simulink model "takeoff"  (R2025b)
settings: Solver=ode4  StartTime=0.0  StopTime=150  FixedStep=0.001  RelTol=1e-3
values from neighbouring files (symbols this model uses):
  a0 = 340.294    [basedata.m]    (also in basedata.mat; control_design.mat; landing_init.m; landing_plan.mat)
  b_ref = 2.0    (= 2)    [basedata.m]    (also in basedata.mat; control_design.mat; landing_init.m; landing_plan.mat)
  c_gear = [0.8e4, 1.4e4, 1.4e4]    [basedata.m]    (also in basedata.mat = [8000 14000 14000]; control_design.mat = [8000 14000 14000]; landing_init.m; landing_plan.mat = [8000 14000 14000])
  c_lat = [1.4e4, 2.2e4, 2.2e4]    [basedata.m]    (also in basedata.mat = [14000 22000 22000]; control_design.mat = [14000 22000 22000]; landing_init.m; landing_plan.mat = [14000 22000 22000])
  c_ref = 0.9    [basedata.m]    (also in basedata.mat; control_design.mat; landing_init.m; landing_plan.mat)
  c_roll = [0.020, 0.018, 0.018]    [basedata.m]    (also in basedata.mat = [0.02 0.018 0.018]; control_design.mat = [0.02 0.018 0.018]; landing_init.m; landing_plan.mat = [0.02 0.018 0.018])
  CD0 = 0.045    [basedata.m]    (also in basedata.mat; canshujisuan.m; control_design.mat; landing_init.m)
  CL0 = 0.083    [basedata.m]    (also in basedata.mat; control_design.mat; landing_init.m; landing_plan.mat)
  CLa = 3.80    (= 3.8)    [basedata.m]    (also in basedata.mat; canshujisuan.m = 2.5; control_design.mat; landing_init.m)
  Clb = -0.08    [basedata.m]    (also in basedata.mat; control_design.mat; landing_init.m; landing_plan.mat)
  Clda = -0.20    (= -0.2)    [basedata.m]    (also in basedata.mat; control_design.mat; landing_init.m; landing_plan.mat)
  CLde = 0.28    [basedata.m]    (also in basedata.mat; control_design.mat; landing_init.m; landing_plan.mat)
  Clp = -0.70    (= -0.7)    [basedata.m]    (also in basedata.mat; control_design.mat; landing_init.m; landing_plan.mat)
  CLq = 4.50    (= 4.5)    [basedata.m]    (also in basedata.mat; canshujisuan.m = 3; control_design.mat; landing_init.m)
  Clr = 0.08    [basedata.m]    (also in basedata.mat; control_design.mat; landing_init.m; landing_plan.mat)
  Cm0 = 0.060    (= 0.06)    [basedata.m]    (also in basedata.mat; control_design.mat; landing_init.m; landing_plan.mat)
  Cma = -0.80    (= -0.8)    [basedata.m]    (also in basedata.mat; control_design.mat; landing_init.m; landing_plan.mat)
  Cmde = -0.90    (= -0.9)    [basedata.m]    (also in basedata.mat; control_design.mat; landing_init.m; landing_plan.mat)
  Cmq = -18.0    (= -18)    [basedata.m]    (also in basedata.mat; control_design.mat; landing_init.m; landing_plan.mat)
  Cnb = 0.25    [basedata.m]    (also in basedata.mat; control_design.mat; landing_init.m; landing_plan.mat)
  Cndr = -0.15    [basedata.m]    (also in basedata.mat; control_design.mat; landing_init.m; landing_plan.mat)
  Cnp = -0.04    [basedata.m]    (also in basedata.mat; control_design.mat; landing_init.m; landing_plan.mat)
  Cnr = -0.45    [basedata.m]    (also in basedata.mat; control_design.mat; landing_init.m; landing_plan.mat)
  CSb = -0.70    (= -0.7)    [basedata.m]    (also in basedata.mat; control_design.mat; landing_init.m; landing_plan.mat)
  CSdr = 0.18    [basedata.m]    (also in basedata.mat; control_design.mat; landing_init.m; landing_plan.mat)
  CSr = 0.12    [basedata.m]    (also in basedata.mat; control_design.mat; landing_init.m; landing_plan.mat)
  D = 0.5 * rho0 * V^2 * S_ref * CD_current    [canshujisuan.m]
  D0 = 1400    [basedata.m]    (also in basedata.mat; control_design.mat; landing.m; landing_init.m)
  da_max = 25    [basedata.m]    (also in basedata.mat; control_design.mat; landing_init.m; landing_plan.mat)
  da_min = -da_max    (= -25)    [basedata.m]    (also in basedata.mat; control_design.mat; landing_init.m; landing_plan.mat)
  de_max = 25    [basedata.m]    (also in basedata.mat; control_design.mat; landing_init.m; landing_plan.mat)
  de_min = -de_max    (= -25)    [basedata.m]    (also in basedata.mat; control_design.mat; landing_init.m; landing_plan.mat)
  DH = pi / 180    (= 0.0174532925199)    [basedata.m]    (also in basedata.mat; control_design.mat; landing_init.m; landing_plan.mat)
  dr_max = 25    [basedata.m]    (also in basedata.mat; control_design.mat; landing_init.m; landing_plan.mat)
  dr_min = -dr_max    (= -25)    [basedata.m]    (also in basedata.mat; control_design.mat; landing_init.m; landing_plan.mat)
  g = 9.80665    [basedata.m]    (also in basedata.mat; canshujisuan.m; control_design.mat; landing_init.m)
  gamma1 = -0.125844364415    [basedata.mat]    (also in landing_trajectory.m = asin(max(min(gamma1_arg, 1), -1)); landingplan.mat)
  gamma2 = -0.0261780104712    [basedata.mat]    (also in landing_trajectory.m = -0.0261799387799; landingplan.mat = 0.0261780104712)
  ground_z = 0.0    (= 0)    [basedata.m]    (also in basedata.mat; control_design.mat; landing_init.m; landing_plan.mat)
  HD = 180 / pi    (= 57.2957795131)    [basedata.m]    (also in basedata.mat; control_design.mat; landing_init.m; landing_plan.mat)
  I = [ Ixx, -Ixy, -Ixz ... (first row only)    [basedata.m]    (also in basedata.mat = [120  0  0; 0  480  0; 0  0  520]; control_design.mat = [120  0  0; 0  480  0; 0  0  520]; landing_init.m; landing_plan.mat = [120  0  0; 0  480  0; 0  0  520])
  K = 0.12    [basedata.m]    (also in basedata.mat; canshujisuan.m = 0.08; control_design.mat; landing_init.m)
  K_alpha = 7.5375    [basedata.mat]    (also in control_design.m = (((wd_pitch^2)-a24))/(2*kesi_pitch*wd_pitch); control_design.mat; controller.m = 5; landingplan.mat)
  k_gear = [1.0e5, 3.0e5, 3.0e5]    [basedata.m]    (also in basedata.mat = [100000 300000 300000]; control_design.mat = [100000 300000 300000]; landing_init.m; landing_plan.mat = [100000 300000 300000])
  Kn_pitch = -0.120095403309    [basedata.mat]    (also in control_design.m = -(2.2*g*(wd_pitch)^2)/(Tr*(((wd_pitch)^2)-a24)*V_control*a34; control_design.mat; controller.m = (2.2*wd^2*g)/(Tr*(wd^2-a24)*V_test*a34); landingplan.mat)
  Kw_pitch = -0.483749055178    [basedata.mat]    (also in control_design.m = -2*kesi_pitch*wd_pitch/a25; control_design.mat; controller.m = -(2*zeta*wd) / a25; landingplan.mat)
  m = 600.0    (= 600)    [basedata.m]    (also in basedata.mat; canshujisuan.m; control_design.mat; landing_init.m)
  mu_brake = [0.0, 0.55, 0.55]    [basedata.m]    (also in basedata.mat = [0 0.55 0.55]; control_design.mat = [0 0.55 0.55]; landing_init.m; landing_plan.mat = [0 0.55 0.55])
  phi0 = 0    [control_design.mat]    (also in landing.m; landing_init.m; landing_init.mat; landing_plan.mat)
  psi0 = 0    [control_design.mat]    (also in landing.m; landing_init.m; landing_init.mat; landing_plan.mat)
  r_left_b = r_gear_b(:,2)    [basedata.m]    (also in basedata.mat = [-0.333333333333 -0.8 0.65]; control_design.mat = [-0.333333333333 -0.8 0.65]; landing_init.m; landing_plan.mat = [-0.333333333333 -0.8 0.65])
  r_nose_b = r_gear_b(:,1)    [basedata.m]    (also in basedata.mat = [2 0 0.65]; control_design.mat = [2 0 0.65]; landing_init.m; landing_plan.mat = [2 0 0.65])
  r_right_b = r_gear_b(:,3)    [basedata.m]    (also in basedata.mat = [-0.333333333333 0.8 0.65]; control_design.mat = [-0.333333333333 0.8 0.65]; landing_init.m; landing_plan.mat = [-0.333333333333 0.8 0.65])
  rho0 = 1.225    [basedata.m]    (also in basedata.mat; canshujisuan.m; control_design.mat; landing_init.m)
  S_ref = 1.2    [basedata.m]    (also in basedata.mat; canshujisuan.m; control_design.mat; landing_init.m)
  theta0 = 0.0523560209424    [control_design.mat]    (also in landing.m = 0; landing_init.m; landing_init.mat = 0.0523598775598; landing_plan.mat)
  u0_b = 128    [control_design.mat]    (also in landing.m; landing_init.m; landing_init.mat = 100; landing_plan.mat)
  v0_b = 0    [control_design.mat]    (also in landing.m; landing_init.m; landing_init.mat; landing_plan.mat)
  v_eps = 0.20    (= 0.2)    [basedata.m]    (also in basedata.mat; control_design.mat; landing_init.m; landing_plan.mat)
  V_min = 3    [control_design.mat]    (also in landing.m; landing_init.m; landing_plan.mat; landingplan.mat)
  w0_b = 0    [control_design.mat]    (also in landing.m; landing_init.m; landing_init.mat; landing_plan.mat)
  wheel_radius = 0.18    [basedata.m]    (also in basedata.mat; control_design.mat; landing_init.m; landing_plan.mat)
  WOW_on = 0.000    (= 0)    [basedata.m]    (also in basedata.mat; control_design.mat; landing_init.m; landing_plan.mat)
  Xg0 = -12000    [control_design.mat]    (also in landing.m; landing_init.m; landing_init.mat = -8000; landing_plan.mat)
  Yg0 = 0    [control_design.mat]    (also in landing.m; landing_init.m; landing_init.mat; landing_plan.mat)
  Zg0 = ground_z - wheel_radius - r_gear_b(3,1) + static_deflection    [basedata.m]    (also in basedata.mat = -0.8215943; control_design.mat = -1000; landing.m = -1000; landing_init.m = -1000)
undefined symbols (not defined in the file or in its folder): I_xz, I_yz, Ix_Iy, Iy_Iz, Iz_Ix
libraries: simulink x52, matrix_library x19
(part 1 of 4)
settings Model: SimulationMode=accelerator  Creator=34355  LastModifiedBy=fjy

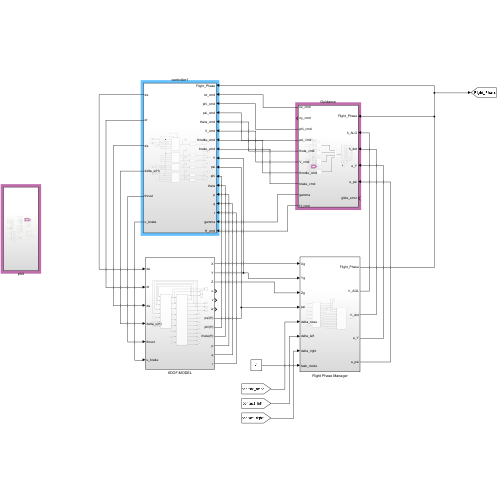
[thumbnail: Simulink's stored preview of the top-level diagram]
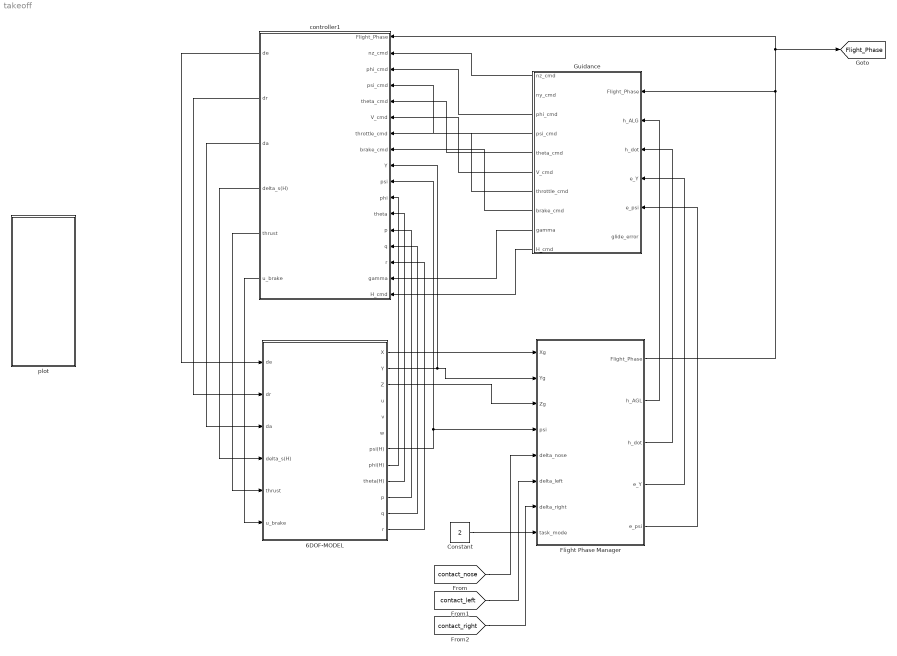
== system takeoff ==
  6DOF-MODEL : Subsystem
  Constant : Constant  Value=2
  Flight Phase Manager : Subsystem
  Guidance : Subsystem
  controller1 : Subsystem
  plot : Subsystem
  tag scope: Flight_Phase=global
  wires:
  Constant/1 -> Flight Phase Manager/8(task_mode)
  6DOF-MODEL/1(X) -> Flight Phase Manager/1(Xg)
  6DOF-MODEL/2(Y) -> Flight Phase Manager/2(Yg), controller1/9(Y)
  6DOF-MODEL/3(Z) -> Flight Phase Manager/3(Zg)
  6DOF-MODEL/7(psi(H)) -> controller1/10(psi), Flight Phase Manager/4(psi)
  [contact_nose] -> Flight Phase Manager/5(delta_nose)
  [contact_left] -> Flight Phase Manager/6(delta_left)
  [contact_right] -> Flight Phase Manager/7(delta_right)
  Flight Phase Manager/1(Flight_Phase) -> controller1/1(Flight_Phase), [Flight_Phase], Guidance/1(Flight_Phase)
  Flight Phase Manager/2(h_AGL) -> Guidance/2(h_ALG)
  Flight Phase Manager/3(h_dot) -> Guidance/3(h_dot)
  Flight Phase Manager/4(e_Y) -> Guidance/4(e_Y)
  Flight Phase Manager/5(e_psi) -> Guidance/5(e_psi)
  Guidance/1(nz_cmd) -> controller1/2(nz_cmd)
  Guidance/3(phi_cmd) -> controller1/3(phi_cmd)
  Guidance/4(psi_cmd) -> controller1/4(psi_cmd)
  Guidance/5(theta_cmd) -> controller1/5(theta_cmd)
  Guidance/6(V_cmd) -> controller1/6(V_cmd)
  Guidance/7(throttle_cmd) -> controller1/7(throttle_cmd)
  Guidance/8(brake_cmd) -> controller1/8(brake_cmd)
  6DOF-MODEL/8(phi(H)) -> controller1/11(phi)
  6DOF-MODEL/9(theta(H)) -> controller1/12(theta)
  6DOF-MODEL/10(p) -> controller1/13(p)
  6DOF-MODEL/11(q) -> controller1/14(q)
  6DOF-MODEL/12(r) -> controller1/15(r)
  controller1/1(de) -> 6DOF-MODEL/1(de)
  controller1/2(dr) -> 6DOF-MODEL/2(dr)
  controller1/3(da) -> 6DOF-MODEL/3(da)
  controller1/4(delta_s(H)) -> 6DOF-MODEL/4(delta_s(H))
  controller1/5(thrust) -> 6DOF-MODEL/5(thrust)
  controller1/6(u_brake) -> 6DOF-MODEL/6(u_brake)
  Guidance/9(gamma) -> controller1/16(gamma)
  Guidance/10(H_cmd) -> controller1/17(H_cmd)

== system takeoff/6DOF-MODEL ==
  de : Inport
  dr : Inport  Port=2
  da : Inport  Port=3
  delta_s(H) : Inport  Port=4
  thrust : Inport  Port=5
  u_brake : Inport  Port=6
  AERO-PARAMETER : Subsystem
  Scope : Scope
      settings: ActiveDisplayYMinimum=1.1177  ActiveDisplayYMaximum=6.98546
  Scope5 : Scope
      settings: ActiveDisplayYMinimum=-8256.02255  ActiveDisplayYMaximum=5856.30436
  Scope6 : Scope
      settings: ActiveDisplayYMinimum=-1607.05651  ActiveDisplayYMaximum=178.56183  DataLoggingVariableName=ScopeData4
  动力学 : Subsystem
  X : Outport
  Y : Outport  Port=2
  Z : Outport  Port=3
  u : Outport  Port=4
  v : Outport  Port=5
  w : Outport  Port=6
  psi(H) : Outport  Port=7
  phi(H) : Outport  Port=8
  theta(H) : Outport  Port=9
  p : Outport  Port=10
  q : Outport  Port=11
  r : Outport  Port=12
  wires:
  动力学/1(alpha(D)) -> Scope/1, AERO-PARAMETER/1(alpha(D))
  thrust/1 -> 动力学/7(thrust)
  u_brake/1 -> 动力学/9(u_brake)
  AERO-PARAMETER/1(D) -> Scope6/1, 动力学/1(D)
  AERO-PARAMETER/2(L) -> Scope5/1, 动力学/2(L)
  AERO-PARAMETER/3(S) -> 动力学/3(S)
  AERO-PARAMETER/4(MX) -> 动力学/4(MX)
  AERO-PARAMETER/5(MY) -> 动力学/5(MY)
  AERO-PARAMETER/6(MZ) -> 动力学/6(MZ)
  delta_s(H)/1 -> 动力学/8(delta_s(H))
  动力学/2(beta(D)) -> AERO-PARAMETER/2(beta(D))
  动力学/3(p) -> p/1, AERO-PARAMETER/3(p(H))
  动力学/4(q) -> q/1, AERO-PARAMETER/4(q(H))
  动力学/5(r) -> r/1, AERO-PARAMETER/5(r(H))
  de/1 -> AERO-PARAMETER/6(de(D))
  dr/1 -> AERO-PARAMETER/7(dr(D))
  da/1 -> AERO-PARAMETER/8(da)
  动力学/14(w) -> w/1
  动力学/7(Y) -> Y/1
  动力学/8(Z) -> Z/1
  动力学/13(v) -> v/1
  动力学/11(psi(H)) -> psi(H)/1
  动力学/12(u) -> u/1
  动力学/10(theta(H)) -> theta(H)/1
  动力学/6(X) -> X/1
  动力学/9(phi(H)) -> phi(H)/1

== system takeoff/Flight Phase Manager ==
  Xg : Inport
  Yg : Inport  Port=2
  Zg : Inport  Port=3
  psi : Inport  Port=4
  delta_nose : Inport  Port=5
  delta_left : Inport  Port=6
  delta_right : Inport  Port=7
  task_mode : Inport  Port=8
  Data Pre-processing : Subsystem
  Phase Logic : Stateflow chart  TreatAsAtomicUnit=on
  Flight_Phase : Outport
  h_AGL : Outport  Port=2
  h_dot : Outport  Port=3
  e_Y : Outport  Port=4
  e_psi : Outport  Port=5
  wires:
  Xg/1 -> Data Pre-processing/1(Xg)
  Yg/1 -> Data Pre-processing/2(Yg)
  Zg/1 -> Data Pre-processing/3(Zg)
  psi/1 -> Data Pre-processing/4(psi)
  delta_nose/1 -> Data Pre-processing/5(delta_nose)
  delta_left/1 -> Data Pre-processing/6(delta_left)
  delta_right/1 -> Data Pre-processing/7(delta_right)
  Phase Logic/1(Flight_Phase) -> Flight_Phase/1
  task_mode/1 -> Phase Logic/13(Task_Mode)
  Data Pre-processing/1(h_AGL) -> h_AGL/1, Phase Logic/1(h_AGL)
  Data Pre-processing/2(V_runway) -> Phase Logic/2(V_runway)
  Data Pre-processing/3(h_dot) -> h_dot/1, Phase Logic/3(h_dot)
  Data Pre-processing/6(nose_on_ground) -> Phase Logic/4(nose_on_ground)
  Data Pre-processing/7(main_on_ground) -> Phase Logic/5(main_on_ground)
  Data Pre-processing/8(airborne) -> Phase Logic/6(airborne)
  Data Pre-processing/9(reach_VR) -> Phase Logic/7(reach_VR)
  Data Pre-processing/10(safe_climb) -> Phase Logic/8(safe_climb)
  Data Pre-processing/11(localizer_captured) -> Phase Logic/9(localizer_captured)
  Data Pre-processing/12(glideslope_captured) -> Phase Logic/10(glideslope_captured)
  Data Pre-processing/13(flare_entry) -> Phase Logic/11(flare_entry)
  Data Pre-processing/14(stop_condition) -> Phase Logic/12(stop_condition)
  Data Pre-processing/4(e_Y) -> e_Y/1
  Data Pre-processing/5(e_psi) -> e_psi/1

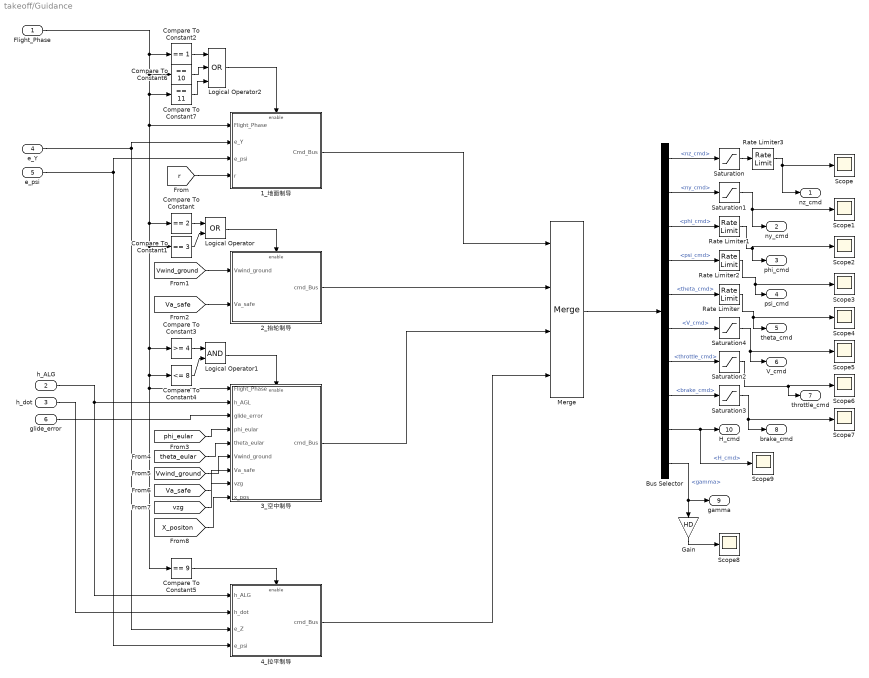
== system takeoff/Guidance ==
  Flight_Phase : Inport
  h_ALG : Inport  Port=2
  h_dot : Inport  Port=3
  e_Y : Inport  Port=4
  e_psi : Inport  Port=5
  glide_error : Inport  Port=6
  1_地面制导 : Subsystem
  "2_抬轮制导 " : Subsystem
  3_空中制导 : Subsystem
  4_拉平制导 : Subsystem
  Bus Selector : BusSelector  OutputSignals=nz_cmd,ny_cmd,phi_cmd,psi_cmd,theta_cmd,V_cmd,throttle_cmd,brake_cmd,H_cmd,gamma
  Compare To Constant : simulink/Logic and Bit Operations/Compare To Constant  relop===  const=2  OutDataTypeStr=boolean
  Compare To Constant1 : simulink/Logic and Bit Operations/Compare To Constant  relop===  const=3  OutDataTypeStr=boolean
  Compare To Constant2 : simulink/Logic and Bit Operations/Compare To Constant  relop===  const=1  OutDataTypeStr=boolean
  Compare To Constant3 : simulink/Logic and Bit Operations/Compare To Constant  relop=>=  const=4  OutDataTypeStr=boolean
  Compare To Constant4 : simulink/Logic and Bit Operations/Compare To Constant  relop=<=  const=8  OutDataTypeStr=boolean
  Compare To Constant5 : simulink/Logic and Bit Operations/Compare To Constant  relop===  const=9  OutDataTypeStr=boolean
  Compare To Constant6 : simulink/Logic and Bit Operations/Compare To Constant  relop===  const=10  OutDataTypeStr=boolean
  Compare To Constant7 : simulink/Logic and Bit Operations/Compare To Constant  relop===  const=11  OutDataTypeStr=boolean
  Gain : Gain  Gain=HD
  Logical Operator : Logic  Operator=OR  AllPortsSameDT=off  OutDataTypeStr=boolean
  Logical Operator1 : Logic  AllPortsSameDT=off  OutDataTypeStr=boolean
  Logical Operator2 : Logic  Operator=OR  Inputs=3  AllPortsSameDT=off  OutDataTypeStr=boolean
  Merge : Merge  Inputs=4
  Rate Limiter : RateLimiter  RisingSlewLimit=1*DH  FallingSlewLimit=-1*DH  SampleTimeMode=inherited
  Rate Limiter1 : RateLimiter  RisingSlewLimit=10*DH  FallingSlewLimit=-10*DH  SampleTimeMode=inherited
  Rate Limiter2 : RateLimiter  RisingSlewLimit=10*DH  FallingSlewLimit=-10*DH  SampleTimeMode=inherited
  Rate Limiter3 : RateLimiter  RisingSlewLimit=0.8  FallingSlewLimit=-0.8  SampleTimeMode=inherited
  Saturation : Saturate  UpperLimit=2  LowerLimit=-2
  Saturation1 : Saturate  UpperLimit=2  LowerLimit=-2
  Saturation2 : Saturate  UpperLimit=1  LowerLimit=0
  Saturation3 : Saturate  UpperLimit=1  LowerLimit=0
  Saturation4 : Saturate  UpperLimit=250  LowerLimit=0
  Scope{,1..9} (10 alike) : Scope
      Scope settings: ActiveDisplayYMinimum=-0.19965  ActiveDisplayYMaximum=1.13329  DataLoggingVariableName=ScopeData2
      Scope1 settings: ActiveDisplayYMinimum=-0.00301  ActiveDisplayYMaximum=0.00493  DataLoggingVariableName=ScopeData3
      Scope2 settings: ActiveDisplayYMinimum=-1  ActiveDisplayYMaximum=1  DataLoggingVariableName=ScopeData4
      Scope3 settings: ActiveDisplayYMinimum=-0.0909  ActiveDisplayYMaximum=0.01814  DataLoggingVariableName=ScopeData5
      Scope4 settings: ActiveDisplayYMinimum=-0.02618  ActiveDisplayYMaximum=0.23562  DataLoggingVariableName=ScopeData6
      Scope5 settings: DataLoggingVariableName=ScopeData7
      Scope6 settings: DataLoggingVariableName=ScopeData8
      Scope7 settings: DataLoggingVariableName=ScopeData9
      Scope8 settings: ActiveDisplayYMinimum=-8.111644826033606  ActiveDisplayYMaximum=0.90129386955928936
      Scope9 settings: ActiveDisplayYMinimum=-113.79263048910924  ActiveDisplayYMaximum=1137.202950532841  DataLoggingVariableName=ScopeData25
  nz_cmd : Outport
  ny_cmd : Outport  Port=2
  phi_cmd : Outport  Port=3
  psi_cmd : Outport  Port=4
  theta_cmd : Outport  Port=5
  V_cmd : Outport  Port=6
  throttle_cmd : Outport  Port=7
  brake_cmd : Outport  Port=8
  gamma : Outport  Port=9
  H_cmd : Outport  Port=10
  wires:
  Flight_Phase/1 -> Compare To Constant6/1, Compare To Constant7/1, 1_地面制导/1(Flight_Phase), Compare To Constant3/1, Compare To Constant4/1, Compare To Constant5/1, 3_空中制导/1(Flight_Phase), Compare To Constant1/1, Compare To Constant/1, Compare To Constant2/1
  e_Y/1 -> 1_地面制导/2(e_Y), 4_拉平制导/3(e_Z)
  Merge/1 -> Bus Selector/1
  e_psi/1 -> 1_地面制导/3(e_psi), 4_拉平制导/4(e_psi)
  h_ALG/1 -> 4_拉平制导/1(h_ALG), 3_空中制导/2(h_AGL)
  h_dot/1 -> 4_拉平制导/2(h_dot)
  glide_error/1 -> 3_空中制导/3(glide_error)
  Saturation1/1 -> ny_cmd/1, Scope1/1
  Compare To Constant/1 -> Logical Operator/1
  Compare To Constant1/1 -> Logical Operator/2
  Logical Operator/1 -> "2_抬轮制导 "/Enable
  Compare To Constant3/1 -> Logical Operator1/1
  Compare To Constant4/1 -> Logical Operator1/2
  Logical Operator1/1 -> 3_空中制导/Enable
  Compare To Constant5/1 -> 4_拉平制导/Enable
  Compare To Constant2/1 -> Logical Operator2/1
  Compare To Constant6/1 -> Logical Operator2/2
  Compare To Constant7/1 -> Logical Operator2/3
  Logical Operator2/1 -> 1_地面制导/Enable
  Rate Limiter/1 -> theta_cmd/1, Scope4/1
  Rate Limiter1/1 -> phi_cmd/1, Scope2/1
  1_地面制导/1(Cmd_Bus) -> Merge/1
  "2_抬轮制导 "/1(cmd_Bus) -> Merge/2
  3_空中制导/1(cmd_Bus) -> Merge/3
  4_拉平制导/1(cmd_Bus) -> Merge/4
  Rate Limiter2/1 -> psi_cmd/1, Scope3/1
  Saturation3/1 -> brake_cmd/1, Scope7/1
  Saturation4/1 -> V_cmd/1, Scope5/1
  Saturation/1 -> Rate Limiter3/1
  Rate Limiter3/1 -> nz_cmd/1, Scope/1
  Saturation2/1 -> throttle_cmd/1, Scope6/1
  [r] -> 1_地面制导/4(r)
  [Vwind_ground] -> "2_抬轮制导 "/1(Vwind_ground)
  [Va_safe] -> "2_抬轮制导 "/2(Va_safe)
  [phi_eular] -> 3_空中制导/4(phi_eular)
  [theta_eular] -> 3_空中制导/5(theta_eular)
  [Vwind_ground] -> 3_空中制导/6(Vwind_ground)
  [Va_safe] -> 3_空中制导/7(Va_safe)
  Bus Selector/1 -> Saturation/1  "<nz_cmd>"
  Bus Selector/2 -> Saturation1/1  "<ny_cmd>"
  Bus Selector/3 -> Rate Limiter1/1  "<phi_cmd>"
  Bus Selector/4 -> Rate Limiter2/1  "<psi_cmd>"
  Bus Selector/5 -> Rate Limiter/1  "<theta_cmd>"
  Bus Selector/6 -> Saturation4/1  "<V_cmd>"
  Bus Selector/7 -> Saturation2/1  "<throttle_cmd>"
  Bus Selector/8 -> Saturation3/1  "<brake_cmd>"
  [vzg] -> 3_空中制导/8(vzg)
  [X_positon] -> 3_空中制导/9(x_pos)
  Bus Selector/10 -> Gain/1, gamma/1  "<gamma>"
  Bus Selector/9 -> Scope9/1, H_cmd/1  "<H_cmd>"
  Gain/1 -> Scope8/1

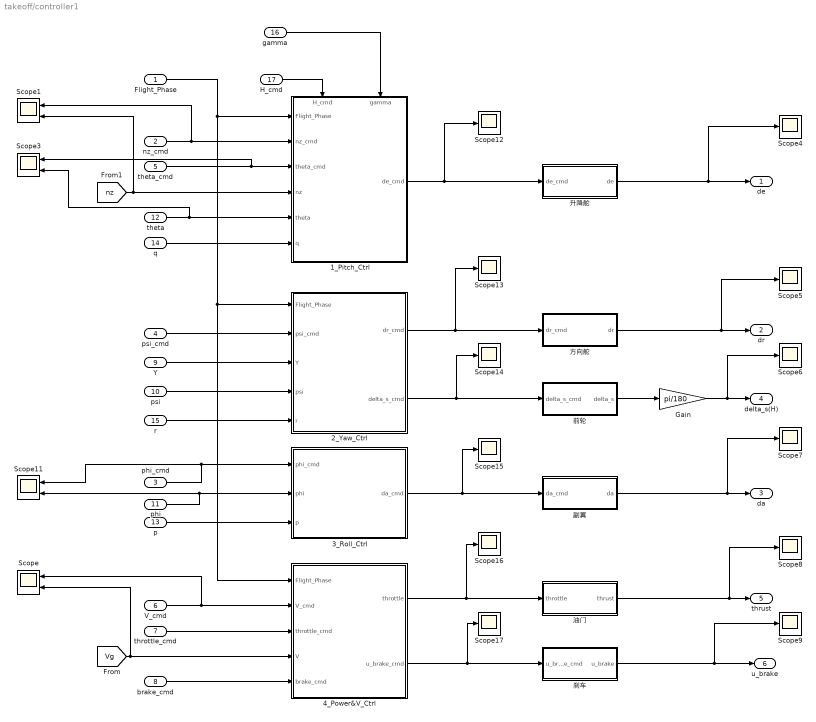
== system takeoff/controller1 ==
  Flight_Phase : Inport
  nz_cmd : Inport  Port=2
  phi_cmd : Inport  Port=3
  psi_cmd : Inport  Port=4
  theta_cmd : Inport  Port=5
  V_cmd : Inport  Port=6
  throttle_cmd : Inport  Port=7
  brake_cmd : Inport  Port=8
  Y : Inport  Port=9
  psi : Inport  Port=10
  phi : Inport  Port=11
  theta : Inport  Port=12
  p : Inport  Port=13
  q : Inport  Port=14
  r : Inport  Port=15
  gamma : Inport  Port=16
  H_cmd : Inport  Port=17
  1_Pitch_Ctrl : Subsystem
      settings: PortSchema="{\"entries\":[{\"content\":{\"sides\":[{\"content\":{\"connectorIds\":[\"In1\",\"In2\",\"In3\",\"In4\",\"In5\",\"In6\"]},\"type\":\"ConnectorPlacement.EquallySpacedRectSide\",\"uuid\":\"27d13232-9f89-4ac1-9c77-5758657de7c7\"},{\"content\":{\"connectorIds\":[\"Out1\"],\"side\":\"RIGHT\"},\"type\":\"ConnectorPlacement.EquallySpacedRectSide\",\"uuid\":\"ae62ad8c-a405-4422-b5ec-9ac723f70591\"},{\"content\":{\"connectorIds\":[\"In7\",\"In8\"],\"side\":\"TOP\"},\"type\":\"ConnectorPlacement.EquallySpacedRectSide\",\"uuid\":\"4cebe0f4-d768-4fb6-931c-2fd4183255b7\"}]},\"type\":\"ConnectorPlacement.EquallySpacedConnector\",\"uuid\":\"2c44e0df-7f94-4dab-9232-216c905b911f\"}],\"packageUris\":[\"http://schema.mathworks.com/mf0/Connector/R2020b\"],\"version\":\"1.0\"}"
  2_Yaw_Ctrl : Subsystem
  3_Roll_Ctrl : Subsystem
  4_Power&V_Ctrl : Subsystem
  Gain : Gain  Gain=pi/180
  Scope{,1,3,11} (4 alike) : Scope  NumInputPorts=2
      Scope settings: ActiveDisplayYMinimum=-25.14963  ActiveDisplayYMaximum=226.34663  DataLoggingVariableName=ScopeData3
      Scope1 settings: ActiveDisplayYMinimum=-0.22546  ActiveDisplayYMaximum=1.36559  DataLoggingVariableName=ScopeData7
      Scope11 settings: ActiveDisplayYMinimum=-0.00059  ActiveDisplayYMaximum=0.00038  DataLoggingVariableName=ScopeData2
      Scope3 settings: ActiveDisplayYMinimum=-0.02682  ActiveDisplayYMaximum=0.23988  DataLoggingVariableName=ScopeData10
  Scope{4..9,12..17} (12 alike) : Scope
      Scope12 settings: ActiveDisplayYMinimum=-14.28559  ActiveDisplayYMaximum=7.54847
      Scope13 settings: ActiveDisplayYMinimum=-7.28617  ActiveDisplayYMaximum=15.25402  DataLoggingVariableName=ScopeData2
      Scope14 settings: ActiveDisplayYMinimum=-0.00117  ActiveDisplayYMaximum=0.0105  DataLoggingVariableName=ScopeData3
      Scope15 settings: ActiveDisplayYMinimum=-0.22974  ActiveDisplayYMaximum=1.237  DataLoggingVariableName=ScopeData4
      Scope16 settings: ActiveDisplayYMinimum=0.24658  ActiveDisplayYMaximum=1.08371  DataLoggingVariableName=ScopeData5
      Scope17 settings: ActiveDisplayYMinimum=-1  ActiveDisplayYMaximum=1  DataLoggingVariableName=ScopeData6
      Scope4 settings: ActiveDisplayYMinimum=-13.80049  ActiveDisplayYMaximum=6.51267  DataLoggingVariableName=ScopeData11
      Scope5 settings: ActiveDisplayYMinimum=-7.23665  ActiveDisplayYMaximum=15.24812
      Scope6 settings: ActiveDisplayYMinimum=-2E-5  ActiveDisplayYMaximum=0.00018  DataLoggingVariableName=ScopeData2
      Scope7 settings: ActiveDisplayYMinimum=-0.15917  ActiveDisplayYMaximum=1.07702  DataLoggingVariableName=ScopeData3
      Scope8 settings: ActiveDisplayYMinimum=-375  ActiveDisplayYMaximum=3375  DataLoggingVariableName=ScopeData4
      Scope9 settings: ActiveDisplayYMinimum=-1  ActiveDisplayYMaximum=1  DataLoggingVariableName=ScopeData5
  刹车 : Subsystem
  前轮 : Subsystem
  副翼 : Subsystem
  升降舵 : Subsystem
  方向舵 : Subsystem
  油门 : Subsystem
  de : Outport
  dr : Outport  Port=2
  da : Outport  Port=3
  delta_s(H) : Outport  Port=4
  thrust : Outport  Port=5
  u_brake : Outport  Port=6
  wires:
  phi_cmd/1 -> Scope11/1, 3_Roll_Ctrl/1(phi_cmd)
  phi/1 -> Scope11/2, 3_Roll_Ctrl/2(phi)
  p/1 -> 3_Roll_Ctrl/3(p)
  brake_cmd/1 -> 4_Power&V_Ctrl/5(brake_cmd)
  4_Power&V_Ctrl/1(throttle) -> 油门/1(throttle), Scope16/1
  Flight_Phase/1 -> 1_Pitch_Ctrl/1(Flight_Phase), 2_Yaw_Ctrl/1(Flight_Phase), 4_Power&V_Ctrl/1(Flight_Phase)
  nz_cmd/1 -> Scope1/1, 1_Pitch_Ctrl/2(nz_cmd)
  psi_cmd/1 -> 2_Yaw_Ctrl/2(psi_cmd)
  [nz] -> Scope1/2, 1_Pitch_Ctrl/4(nz)
  q/1 -> 1_Pitch_Ctrl/6(q)
  V_cmd/1 -> Scope/1, 4_Power&V_Ctrl/2(V_cmd)
  [Vg] -> Scope/2, 4_Power&V_Ctrl/4(V)
  Gain/1 -> Scope6/1, delta_s(H)/1
  theta_cmd/1 -> Scope3/1, 1_Pitch_Ctrl/3(theta_cmd)
  1_Pitch_Ctrl/1(de_cmd) -> 升降舵/1(de_cmd), Scope12/1
  2_Yaw_Ctrl/1(dr_cmd) -> Scope13/1, 方向舵/1(dr_cmd)
  2_Yaw_Ctrl/2(delta_s_cmd) -> Scope14/1, 前轮/1(delta_s_cmd)
  3_Roll_Ctrl/1(da_cmd) -> Scope15/1, 副翼/1(da_cmd)
  4_Power&V_Ctrl/2(u_brake_cmd) -> 刹车/1(u_brake_cmd), Scope17/1
  theta/1 -> Scope3/2, 1_Pitch_Ctrl/5(theta)
  throttle_cmd/1 -> 4_Power&V_Ctrl/3(throttle_cmd)
  Y/1 -> 2_Yaw_Ctrl/3(Y)
  psi/1 -> 2_Yaw_Ctrl/4(psi)
  r/1 -> 2_Yaw_Ctrl/5(r)
  升降舵/1(de) -> Scope4/1, de/1
  方向舵/1(dr) -> Scope5/1, dr/1
  前轮/1(delta_s) -> Gain/1
  副翼/1(da) -> Scope7/1, da/1
  油门/1(thrust) -> Scope8/1, thrust/1
  刹车/1(u_brake) -> Scope9/1, u_brake/1
  H_cmd/1 -> 1_Pitch_Ctrl/7(H_cmd)
  gamma/1 -> 1_Pitch_Ctrl/8(gamma)

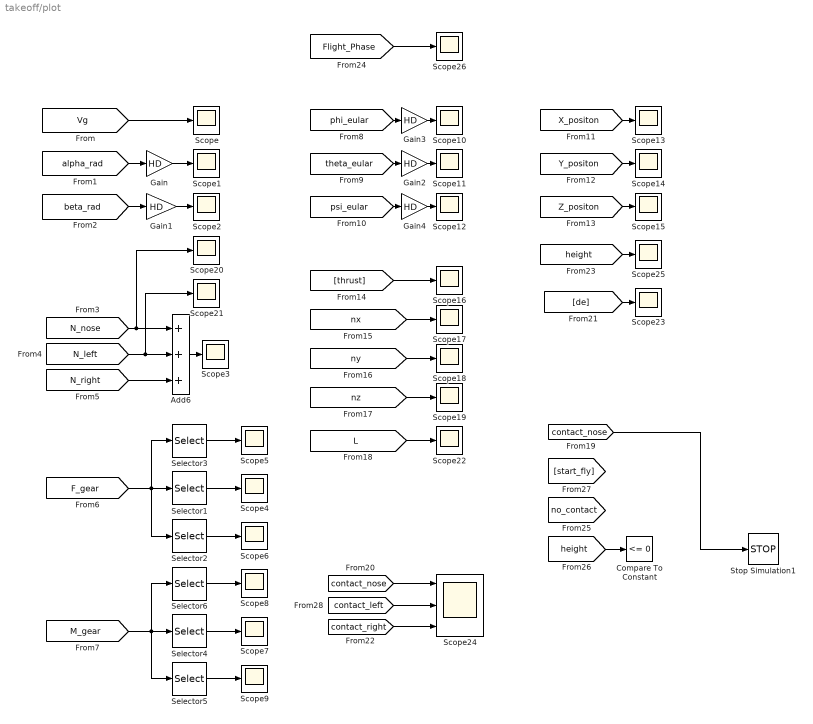
== system takeoff/plot ==
  Add6 : Sum  Inputs=+++
  Compare To Constant : simulink/Logic and Bit Operations/Compare To Constant  relop=<=  const=0  OutDataTypeStr=boolean
  Gain{,1..4} (5 alike) : Gain  Gain=HD
  Scope{,1..23,25..26} (26 alike) : Scope
      Scope settings: ActiveDisplayYMinimum=118.60732407894886  ActiveDisplayYMaximum=211.43694512925961
      Scope1 settings: ActiveDisplayYMinimum=-66.97288  ActiveDisplayYMaximum=12.39263  DataLoggingVariableName=ScopeData2
      Scope10 settings: ActiveDisplayYMinimum=-0.02449  ActiveDisplayYMaximum=0.1104  DataLoggingVariableName=ScopeData12
      Scope11 settings: ActiveDisplayYMinimum=-8.03156734153454  ActiveDisplayYMaximum=9.991113407153664  DataLoggingVariableName=ScopeData13
      Scope12 settings: ActiveDisplayYMinimum=-2.0624  ActiveDisplayYMaximum=0.22916  DataLoggingVariableName=ScopeData14
      Scope13 settings: ActiveDisplayYMinimum=-457.52925  ActiveDisplayYMaximum=4117.76325  DataLoggingVariableName=ScopeData15
      Scope14 settings: ActiveDisplayYMinimum=-1.79752  ActiveDisplayYMaximum=0.19975  DataLoggingVariableName=ScopeData16
      Scope15 settings: ActiveDisplayYMinimum=-1124.98258  ActiveDisplayYMaximum=124.08518  DataLoggingVariableName=ScopeData17
      Scope16 settings: ActiveDisplayYMinimum=1428.28526  ActiveDisplayYMaximum=3174.63497  DataLoggingVariableName=ScopeData18
      Scope17 settings: ActiveDisplayYMinimum=-0.69402  ActiveDisplayYMaximum=5.48306  DataLoggingVariableName=ScopeData19
      Scope18 settings: ActiveDisplayYMinimum=-1  ActiveDisplayYMaximum=1  DataLoggingVariableName=ScopeData20
      Scope19 settings: ActiveDisplayYMinimum=-1.39533  ActiveDisplayYMaximum=-0.75578  DataLoggingVariableName=ScopeData21
      Scope2 settings: ActiveDisplayYMinimum=-0.24043  ActiveDisplayYMaximum=0.0115  DataLoggingVariableName=ScopeData3
      Scope20 settings: ActiveDisplayYMinimum=-109.07344  ActiveDisplayYMaximum=981.66096  DataLoggingVariableName=ScopeData2
      Scope21 settings: ActiveDisplayYMinimum=-315.21375  ActiveDisplayYMaximum=2836.92375  DataLoggingVariableName=ScopeData5
      Scope22 settings: ActiveDisplayYMinimum=-1.39533  ActiveDisplayYMaximum=-0.75578  DataLoggingVariableName=ScopeData5
      Scope23 settings: ActiveDisplayYMinimum=-4.93736  ActiveDisplayYMaximum=28.32637
      Scope25 settings: ActiveDisplayYMinimum=-125.13549679187696  ActiveDisplayYMaximum=1136.7614641690736
      Scope26 settings: ActiveDisplayYMinimum=5.75  ActiveDisplayYMaximum=8.25  DataLoggingVariableName=ScopeData4
      Scope3 settings: ActiveDisplayYMinimum=-6.8710410861604161E+86  ActiveDisplayYMaximum=6.1839369775443757E+87  DataLoggingVariableName=ScopeData4
      Scope4 settings: ActiveDisplayYMinimum=-1  ActiveDisplayYMaximum=1  DataLoggingVariableName=ScopeData6
      Scope5 settings: ActiveDisplayYMinimum=-126.98754  ActiveDisplayYMaximum=57.45616  DataLoggingVariableName=ScopeData7
      Scope6 settings: ActiveDisplayYMinimum=-6622.10957  ActiveDisplayYMaximum=735.78995  DataLoggingVariableName=ScopeData8
      Scope7 settings: ActiveDisplayYMinimum=5883.9899999999234  ActiveDisplayYMaximum=5883.99000000002  DataLoggingVariableName=ScopeData9
      Scope8 settings: ActiveDisplayYMinimum=-1  ActiveDisplayYMaximum=1  DataLoggingVariableName=ScopeData10
      Scope9 settings: ActiveDisplayYMinimum=-1  ActiveDisplayYMaximum=1  DataLoggingVariableName=ScopeData11
  Scope24 : Scope  NumInputPorts=3
      settings: ActiveDisplayYMinimum=-0.125  ActiveDisplayYMaximum=1.125  DataLoggingVariableName=ScopeData6
  Selector1 : Selector  InputPortWidth=3  IndexOptions=Index vector (dialog)  Indices=2  OutputSizes=1
  Selector2 : Selector  InputPortWidth=3  IndexOptions=Index vector (dialog)  Indices=3  OutputSizes=1
  Selector3 : Selector  InputPortWidth=3  IndexOptions=Index vector (dialog)  Indices=1  OutputSizes=1
  Selector4 : Selector  InputPortWidth=3  IndexOptions=Index vector (dialog)  Indices=2  OutputSizes=1
  Selector5 : Selector  InputPortWidth=3  IndexOptions=Index vector (dialog)  Indices=3  OutputSizes=1
  Selector6 : Selector  InputPortWidth=3  IndexOptions=Index vector (dialog)  Indices=1  OutputSizes=1
  Stop Simulation1 : Stop
  wires:
  [N_nose] -> Add6/1, Scope20/1
  [N_left] -> Scope21/1, Add6/2
  [N_right] -> Add6/3
  [Vg] -> Scope/1
  [alpha_rad] -> Gain/1
  [beta_rad] -> Gain1/1
  Add6/1 -> Scope3/1
  Selector3/1 -> Scope5/1
  Selector2/1 -> Scope6/1
  Selector1/1 -> Scope4/1
  [F_gear] -> Selector2/1, Selector1/1, Selector3/1
  Selector6/1 -> Scope8/1
  Selector4/1 -> Scope7/1
  [M_gear] -> Selector6/1, Selector4/1, Selector5/1
  Selector5/1 -> Scope9/1
  [psi_eular] -> Gain4/1
  [theta_eular] -> Gain2/1
  [phi_eular] -> Gain3/1
  Gain1/1 -> Scope2/1
  Gain/1 -> Scope1/1
  Gain2/1 -> Scope11/1
  [Y_positon] -> Scope14/1
  [X_positon] -> Scope13/1
  [Z_positon] -> Scope15/1
  Gain3/1 -> Scope10/1
  Gain4/1 -> Scope12/1
  [thrust] -> Scope16/1
  [nx] -> Scope17/1
  [ny] -> Scope18/1
  [nz] -> Scope19/1
  [L] -> Scope22/1
  [de] -> Scope23/1
  [contact_nose] -> Stop Simulation1/1
  [height] -> Scope25/1
  [height] -> Compare To Constant/1
  [contact_nose] -> Scope24/1
  [contact_left] -> Scope24/2
  [contact_right] -> Scope24/3
  [Flight_Phase] -> Scope26/1

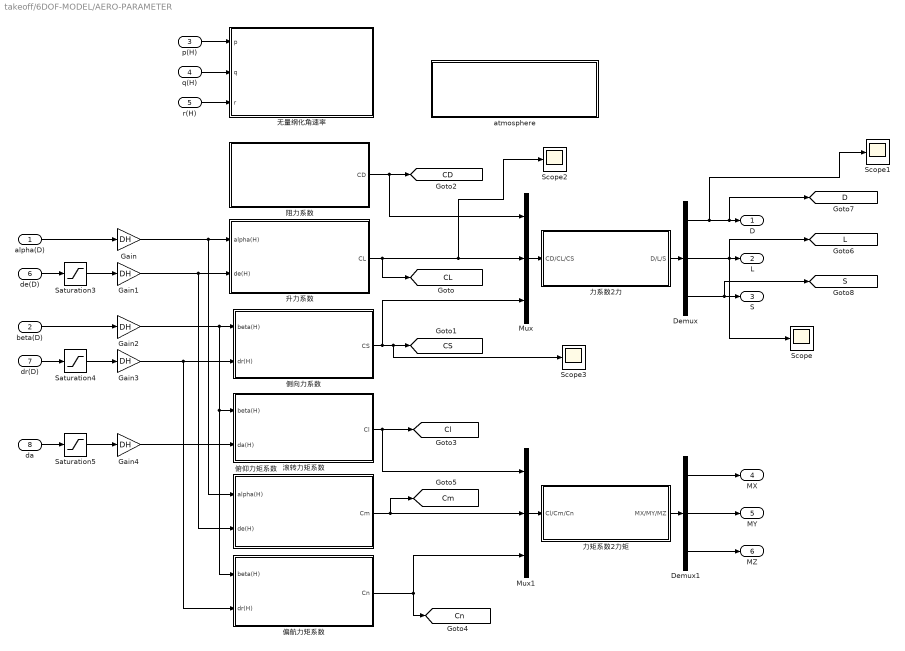
== system takeoff/6DOF-MODEL/AERO-PARAMETER ==
  alpha(D) : Inport
  beta(D) : Inport  Port=2
  p(H) : Inport  Port=3
  q(H) : Inport  Port=4
  r(H) : Inport  Port=5
  de(D) : Inport  Port=6
  dr(D) : Inport  Port=7
  da : Inport  Port=8
  Demux : Demux  Outputs=3
  Demux1 : Demux  Outputs=3
  Gain{,1..4} (5 alike) : Gain  Gain=DH
  Mux : Mux  Inputs=3
  Mux1 : Mux  Inputs=3
  Saturation3 : Saturate  UpperLimit=de_max  LowerLimit=de_min
  Saturation4 : Saturate  UpperLimit=dr_max  LowerLimit=dr_min
  Saturation5 : Saturate  UpperLimit=da_max  LowerLimit=da_min
  Scope{,1..3} (4 alike) : Scope
      Scope settings: ActiveDisplayYMinimum=-8344.45381  ActiveDisplayYMaximum=927.16153  DataLoggingVariableName=ScopeData20
      Scope1 settings: ActiveDisplayYMinimum=568.90057  ActiveDisplayYMaximum=1072.36921  DataLoggingVariableName=ScopeData24
      Scope2 settings: ActiveDisplayYMinimum=-7.3517  ActiveDisplayYMaximum=7.03431  DataLoggingVariableName=ScopeData2
      Scope3 settings: ActiveDisplayYMinimum=-0.27324  ActiveDisplayYMaximum=0.20902  DataLoggingVariableName=ScopeData2
  atmosphere : Subsystem
  侧向力系数 : Subsystem
  俯仰力矩系数 : Subsystem
  偏航力矩系数 : Subsystem
  力矩系数2力矩 : Subsystem
  力系数2力 : Subsystem
  升力系数 : Subsystem
  无量纲化角速率 : Subsystem
  滚转力矩系数 : Subsystem
  阻力系数 : Subsystem
  D : Outport
  L : Outport  Port=2
  S : Outport  Port=3
  MX : Outport  Port=4
  MY : Outport  Port=5
  MZ : Outport  Port=6
  tag scope: CD=global, CL=global, CS=global, Cl=global, Cm=global, Cn=global, D=global, L=global, S=global
  wires:
  升力系数/1(CL) -> [CL], Scope2/1, Mux/2
  侧向力系数/1(CS) -> Mux/3, Scope3/1, [CS]
  da/1 -> Saturation5/1
  Saturation5/1 -> Gain4/1
  Saturation4/1 -> Gain3/1
  dr(D)/1 -> Saturation4/1
  de(D)/1 -> Saturation3/1
  Saturation3/1 -> Gain1/1
  beta(D)/1 -> Gain2/1
  alpha(D)/1 -> Gain/1
  Gain/1 -> 升力系数/1(alpha(H)), 俯仰力矩系数/1(alpha(H))
  Gain1/1 -> 升力系数/2(de(H)), 俯仰力矩系数/2(de(H))
  Gain2/1 -> 侧向力系数/1(beta(H)), 偏航力矩系数/1(beta(H)), 滚转力矩系数/1(beta(H))
  Gain3/1 -> 侧向力系数/2(dr(H)), 偏航力矩系数/2(dr(H))
  Gain4/1 -> 滚转力矩系数/2(da(H))
  p(H)/1 -> 无量纲化角速率/1(p)
  q(H)/1 -> 无量纲化角速率/2(q)
  r(H)/1 -> 无量纲化角速率/3(r)
  阻力系数/1(CD) -> Mux/1, [CD]
  滚转力矩系数/1(Cl) -> [Cl], Mux1/1
  俯仰力矩系数/1(Cm) -> Mux1/2, [Cm]
  偏航力矩系数/1(Cn) -> [Cn], Mux1/3
  Mux/1 -> 力系数2力/1(CD/CL/CS)
  Mux1/1 -> 力矩系数2力矩/1(Cl/Cm/Cn)
  Demux/2 -> Scope/1, [L], L/1
  力系数2力/1(D/L/S) -> Demux/1
  Demux/1 -> Scope1/1, [D], D/1
  Demux/3 -> [S], S/1
  力矩系数2力矩/1(MX/MY/MZ) -> Demux1/1
  Demux1/1 -> MX/1
  Demux1/2 -> MY/1
  Demux1/3 -> MZ/1

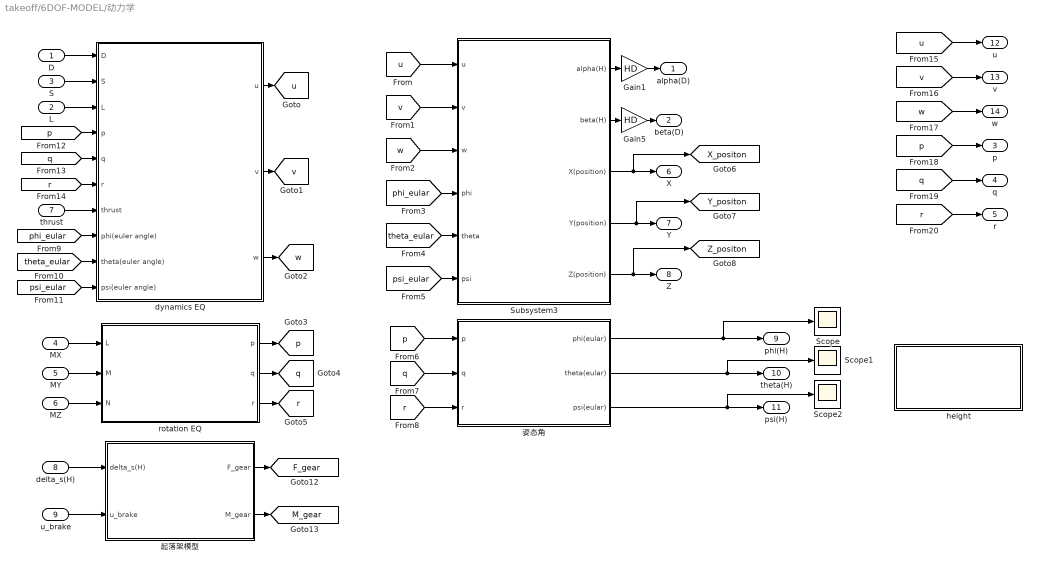
== system takeoff/6DOF-MODEL/动力学 ==
  D : Inport
  L : Inport  Port=2
  S : Inport  Port=3
  MX : Inport  Port=4
  MY : Inport  Port=5
  MZ : Inport  Port=6
  thrust : Inport  Port=7
  delta_s(H) : Inport  Port=8
  u_brake : Inport  Port=9
  Gain1 : Gain  Gain=HD
  Gain5 : Gain  Gain=HD
  Scope : Scope
      settings: ActiveDisplayYMinimum=-1  ActiveDisplayYMaximum=1  DataLoggingVariableName=ScopeData4
  Scope1 : Scope
      settings: ActiveDisplayYMinimum=-57.279  ActiveDisplayYMaximum=136.57236  DataLoggingVariableName=ScopeData5
  Scope2 : Scope
      settings: ActiveDisplayYMinimum=-12.64721  ActiveDisplayYMaximum=113.82488  DataLoggingVariableName=ScopeData6
  Subsystem3 : Subsystem
  dynamics EQ : Subsystem
  height : Subsystem
  rotation EQ : Subsystem
  姿态角 : Subsystem
  起落架模型 : Subsystem
  alpha(D) : Outport
  beta(D) : Outport  Port=2
  p : Outport  Port=3
  q : Outport  Port=4
  r : Outport  Port=5
  X : Outport  Port=6
  Y : Outport  Port=7
  Z : Outport  Port=8
  phi(H) : Outport  Port=9
  theta(H) : Outport  Port=10
  psi(H) : Outport  Port=11
  u : Outport  Port=12
  v : Outport  Port=13
  w : Outport  Port=14
  tag scope: F_gear=global, M_gear=global, X_positon=global, Y_positon=global, Z_positon=global, p=global, q=global, r=global, u=global, v=global, w=global
  wires:
  姿态角/1(phi(eular)) -> Scope/1, phi(H)/1
  姿态角/2(theta(eular)) -> theta(H)/1, Scope1/1
  姿态角/3(psi(eular)) -> psi(H)/1, Scope2/1
  Gain5/1 -> beta(D)/1
  Gain1/1 -> alpha(D)/1
  [u] -> u/1
  [v] -> v/1
  [w] -> w/1
  [p] -> p/1
  [q] -> q/1
  [r] -> r/1
  起落架模型/1(F_gear) -> [F_gear]
  起落架模型/2(M_gear) -> [M_gear]
  MX/1 -> rotation EQ/1(L)
  MY/1 -> rotation EQ/2(M)
  MZ/1 -> rotation EQ/3(N)
  D/1 -> dynamics EQ/1(D)
  S/1 -> dynamics EQ/2(S)
  L/1 -> dynamics EQ/3(L)
  [p] -> dynamics EQ/4(p)
  [q] -> dynamics EQ/5(q)
  [r] -> dynamics EQ/6(r)
  thrust/1 -> dynamics EQ/7(thrust)
  [phi_eular] -> dynamics EQ/8(phi(euler angle))
  [theta_eular] -> dynamics EQ/9(theta(euler angle))
  [psi_eular] -> dynamics EQ/10(psi(euler angle))
  dynamics EQ/1(u) -> [u]
  dynamics EQ/2(v) -> [v]
  dynamics EQ/3(w) -> [w]
  [u] -> Subsystem3/1(u)
  [v] -> Subsystem3/2(v)
  [w] -> Subsystem3/3(w)
  [phi_eular] -> Subsystem3/4(phi)
  [theta_eular] -> Subsystem3/5(theta)
  [psi_eular] -> Subsystem3/6(psi)
  Subsystem3/1(alpha(H)) -> Gain1/1
  Subsystem3/2(beta(H)) -> Gain5/1
  Subsystem3/3(X(position)) -> [X_positon], X/1
  Subsystem3/4(Y(position)) -> [Y_positon], Y/1
  Subsystem3/5(Z(position)) -> [Z_positon], Z/1
  delta_s(H)/1 -> 起落架模型/1(delta_s(H))
  u_brake/1 -> 起落架模型/2(u_brake)
  rotation EQ/1(p) -> [p]
  rotation EQ/2(q) -> [q]
  rotation EQ/3(r) -> [r]
  [p] -> 姿态角/1(p)
  [q] -> 姿态角/2(q)
  [r] -> 姿态角/3(r)

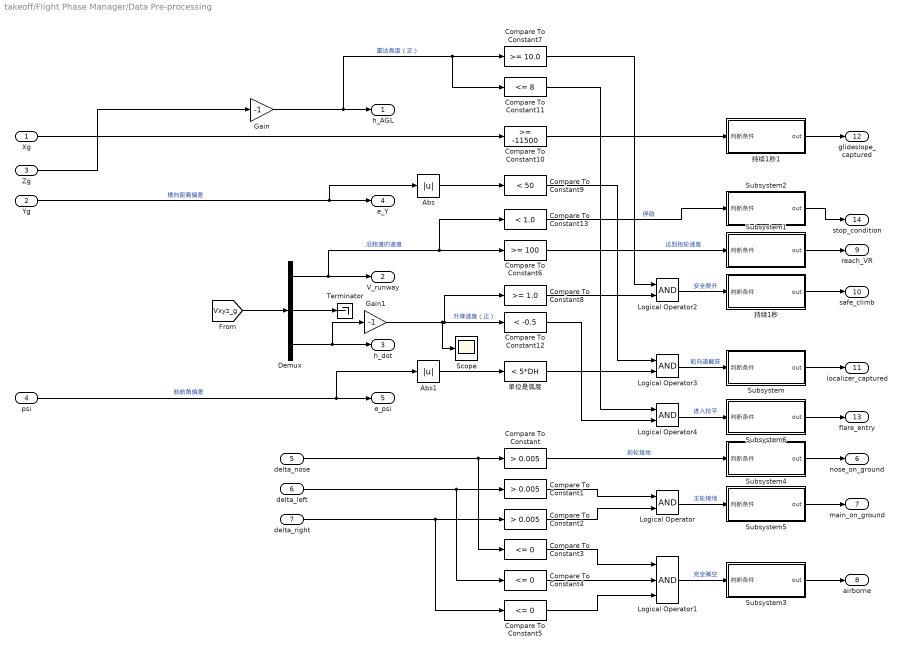
== system takeoff/Flight Phase Manager/Data Pre-processing ==
  Xg : Inport
  Yg : Inport  Port=2
  Zg : Inport  Port=3
  psi : Inport  Port=4
  delta_nose : Inport  Port=5
  delta_left : Inport  Port=6
  delta_right : Inport  Port=7
  Abs : Abs  SaturateOnIntegerOverflow=off
  Abs1 : Abs  SaturateOnIntegerOverflow=off
  Compare To Constant : simulink/Logic and Bit Operations/Compare To Constant  relop=>  const=0.005  OutDataTypeStr=boolean
  Compare To Constant1 : simulink/Logic and Bit Operations/Compare To Constant  relop=>  const=0.005  OutDataTypeStr=boolean
  Compare To Constant10 : simulink/Logic and Bit Operations/Compare To Constant  relop=>=  const=-11500  OutDataTypeStr=boolean
  Compare To Constant11 : simulink/Logic and Bit Operations/Compare To Constant  relop=<=  const=8  OutDataTypeStr=boolean
  Compare To Constant12 : simulink/Logic and Bit Operations/Compare To Constant  relop=<  const=-0.5  OutDataTypeStr=boolean
  Compare To Constant13 : simulink/Logic and Bit Operations/Compare To Constant  relop=<  const=1.0  OutDataTypeStr=boolean
  Compare To Constant2 : simulink/Logic and Bit Operations/Compare To Constant  relop=>  const=0.005  OutDataTypeStr=boolean
  Compare To Constant3 : simulink/Logic and Bit Operations/Compare To Constant  relop=<=  const=0  OutDataTypeStr=boolean
  Compare To Constant4 : simulink/Logic and Bit Operations/Compare To Constant  relop=<=  const=0  OutDataTypeStr=boolean
  Compare To Constant5 : simulink/Logic and Bit Operations/Compare To Constant  relop=<=  const=0  OutDataTypeStr=boolean
  Compare To Constant6 : simulink/Logic and Bit Operations/Compare To Constant  relop=>=  const=100  OutDataTypeStr=boolean
  Compare To Constant7 : simulink/Logic and Bit Operations/Compare To Constant  relop=>=  const=10.0  OutDataTypeStr=boolean
  Compare To Constant8 : simulink/Logic and Bit Operations/Compare To Constant  relop=>=  const=1.0  OutDataTypeStr=boolean
  Compare To Constant9 : simulink/Logic and Bit Operations/Compare To Constant  relop=<  const=50  OutDataTypeStr=boolean
  Demux : Demux  Outputs=3
  Gain : Gain  Gain=-1
  Gain1 : Gain  Gain=-1
  Logical Operator{,2..4} (4 alike) : Logic  AllPortsSameDT=off  OutDataTypeStr=boolean
  Logical Operator1 : Logic  Inputs=3  AllPortsSameDT=off  OutDataTypeStr=boolean
  Scope : Scope
      settings: ActiveDisplayYMinimum=-23.10985  ActiveDisplayYMaximum=40.49102  DataLoggingVariableName=ScopeData5
  Subsystem : Subsystem
  Subsystem1 : Subsystem
  Subsystem2 : Subsystem
  Subsystem3 : Subsystem
  Subsystem4 : Subsystem
  Subsystem5 : Subsystem
  Subsystem6 : Subsystem
  Terminator : Terminator
  单位是弧度 : simulink/Logic and Bit Operations/Compare To Constant  relop=<  const=5*DH  OutDataTypeStr=boolean
  持续1秒 : Subsystem
  持续1秒1 : Subsystem
  h_AGL : Outport
  V_runway : Outport  Port=2
  h_dot : Outport  Port=3
  e_Y : Outport  Port=4
  e_psi : Outport  Port=5
  nose_on_ground : Outport  Port=6
  main_on_ground : Outport  Port=7
  airborne : Outport  Port=8
  reach_VR : Outport  Port=9
  safe_climb : Outport  Port=10
  localizer_captured : Outport  Port=11
  glideslope_captured : Outport  Port=12
  flare_entry : Outport  Port=13
  stop_condition : Outport  Port=14
  wires:
  [Vxyz_g] -> Demux/1
  Demux/1 -> V_runway/1, Compare To Constant13/1, Compare To Constant6/1  "沿跑道的速度"
  psi/1 -> e_psi/1, Abs1/1  "航航角偏差"
  delta_nose/1 -> Compare To Constant3/1, Compare To Constant/1
  delta_left/1 -> Compare To Constant1/1, Compare To Constant4/1
  delta_right/1 -> Compare To Constant2/1, Compare To Constant5/1
  Compare To Constant1/1 -> Logical Operator/1
  Compare To Constant2/1 -> Logical Operator/2
  Compare To Constant4/1 -> Logical Operator1/2
  Compare To Constant3/1 -> Logical Operator1/1
  Compare To Constant5/1 -> Logical Operator1/3
  Compare To Constant8/1 -> Logical Operator2/2
  Compare To Constant7/1 -> Logical Operator2/1
  Abs/1 -> Compare To Constant9/1
  Abs1/1 -> 单位是弧度/1
  单位是弧度/1 -> Logical Operator3/2
  Compare To Constant9/1 -> Logical Operator3/1
  Compare To Constant11/1 -> Logical Operator4/1
  Compare To Constant12/1 -> Logical Operator4/2
  持续1秒/1(out) -> safe_climb/1
  Logical Operator3/1 -> Subsystem/1(判断条件)  "航向道截获"
  Subsystem/1(out) -> localizer_captured/1
  Logical Operator2/1 -> 持续1秒/1(判断条件)  "安全爬升"
  持续1秒1/1(out) -> glideslope_captured/1
  Subsystem1/1(out) -> reach_VR/1
  Compare To Constant6/1 -> Subsystem1/1(判断条件)  "达到抬轮速度"
  Subsystem2/1(out) -> stop_condition/1
  Compare To Constant13/1 -> Subsystem2/1(判断条件)  "停稳"
  Logical Operator1/1 -> Subsystem3/1(判断条件)  "完全腾空"
  Subsystem3/1(out) -> airborne/1
  Subsystem4/1(out) -> nose_on_ground/1
  Compare To Constant/1 -> Subsystem4/1(判断条件)  "前轮接地"
  Subsystem5/1(out) -> main_on_ground/1
  Logical Operator/1 -> Subsystem5/1(判断条件)  "主轮接地"
  Subsystem6/1(out) -> flare_entry/1
  Logical Operator4/1 -> Subsystem6/1(判断条件)  "进入拉平"
  Zg/1 -> Gain/1
  Yg/1 -> e_Y/1, Abs/1  "横向距离偏差"
  Gain/1 -> h_AGL/1, Compare To Constant7/1, Compare To Constant11/1  "雷达高度（正）"
  Gain1/1 -> Scope/1, Compare To Constant8/1, Compare To Constant12/1  "升降速度（正）"
  Demux/2 -> Terminator/1
  Demux/3 -> Gain1/1, h_dot/1
  Compare To Constant10/1 -> 持续1秒1/1(判断条件)
  Xg/1 -> Compare To Constant10/1

== system takeoff/Guidance/1_地面制导 ==
  Flight_Phase : Inport
  e_Y : Inport  Port=2
  e_psi : Inport  Port=3
  r : Inport  Port=4
  Enable : EnablePort
  Bus Creator : BusCreator  Inputs=10
  Compare To Constant1 : simulink/Logic and Bit Operations/Compare To Constant  relop===  const=11  OutDataTypeStr=boolean
  Constant : Constant  Value=0
  Constant3 : Constant
  Gain : Gain  Gain=-1
  Gain2 : Gain  Gain=0.08
  Gain3 : Gain  Gain=-0.85
  Gain4 : Gain  Gain=-0.2
  H_cmd : Constant  Value=0
  Sum : Sum  Inputs=|++
  Sum1 : Sum  Inputs=|++
  Switch1 : Switch  Criteria=u2 > Threshold  SaturateOnIntegerOverflow=off  InputSameDT=off
  V_cmd : Constant  Value=0
  gamma : Constant  Value=0
  ny_cmd : Constant  Value=0.0
  nz_cmd : Constant  Value=1.0
  phi_cmd : Constant  Value=0.0
  psi_cmd : Saturate  UpperLimit=25*pi/180  LowerLimit=-25*pi/180
  theta_cmd : Constant  Value=0.0
  throttle_cmd : Constant
  Cmd_Bus : Outport
  wires:
  Flight_Phase/1 -> Compare To Constant1/1
  Compare To Constant1/1 -> Switch1/2
  Constant3/1 -> Switch1/1
  Constant/1 -> Switch1/3
  nz_cmd/1 -> Bus Creator/1  "nz_cmd"
  ny_cmd/1 -> Bus Creator/2  "ny_cmd"
  phi_cmd/1 -> Bus Creator/3  "phi_cmd"
  psi_cmd/1 -> Bus Creator/4  "psi_cmd"
  theta_cmd/1 -> Bus Creator/5  "theta_cmd"
  Switch1/1 -> Bus Creator/8  "brake_cmd"
  Bus Creator/1 -> Cmd_Bus/1
  e_Y/1 -> Gain/1
  throttle_cmd/1 -> Bus Creator/7  "throttle_cmd"
  Gain/1 -> Gain2/1
  e_psi/1 -> Gain3/1
  Gain2/1 -> Sum/1
  Gain3/1 -> Sum/2
  Sum/1 -> Sum1/1
  Gain4/1 -> Sum1/2
  Sum1/1 -> psi_cmd/1
  V_cmd/1 -> Bus Creator/6  "V_cmd"
  r/1 -> Gain4/1
  gamma/1 -> Bus Creator/9  "gamma"
  H_cmd/1 -> Bus Creator/10  "H_cmd"

== system takeoff/Guidance/2_抬轮制导  ==
  Vwind_ground : Inport
  Va_safe : Inport  Port=2
  Enable : EnablePort  StatesWhenEnabling=reset
  Asin : Trigonometry  Operator=asin
  Bus Creator : BusCreator  Inputs=10
  Constant : Constant  Value=12
  Constant1 : Constant  Value=0
  Divide : Product  Inputs=*/
  Gain : Gain  Gain=DH
  Gain1 : Gain  Gain=-1
  H_cmd : Constant  Value=0
  Saturation2 : Saturate  UpperLimit=10*DH  LowerLimit=-10*DH
  Selector : Selector  InputPortWidth=3  IndexOptions=Index vector (dialog)  Indices=2  OutputSizes=1
  V_cmd : Constant  Value=200
  gamma : Constant  Value=0
  ny_cmd : Constant  Value=0
  nz_cmd : Constant
  phi_cmd : Constant  Value=0
  throttle_cmd : Constant
  cmd_Bus : Outport  InitialOutput=0
  wires:
  Constant1/1 -> Bus Creator/8  "brake_cmd"
  Saturation2/1 -> Bus Creator/4  "psi_cmd"
  V_cmd/1 -> Bus Creator/6  "V_cmd"
  throttle_cmd/1 -> Bus Creator/7  "throttle_cmd"
  nz_cmd/1 -> Bus Creator/1  "nz_cmd"
  Gain/1 -> Bus Creator/5  "theta_cmd"
  ny_cmd/1 -> Bus Creator/2  "ny_cmd"
  Bus Creator/1 -> cmd_Bus/1
  phi_cmd/1 -> Bus Creator/3  "phi_cmd"
  Constant/1 -> Gain/1
  Gain1/1 -> Saturation2/1
  Selector/1 -> Divide/1
  Divide/1 -> Asin/1
  Asin/1 -> Gain1/1
  Va_safe/1 -> Divide/2
  Vwind_ground/1 -> Selector/1
  H_cmd/1 -> Bus Creator/10  "H_cmd"
  gamma/1 -> Bus Creator/9  "gamma"

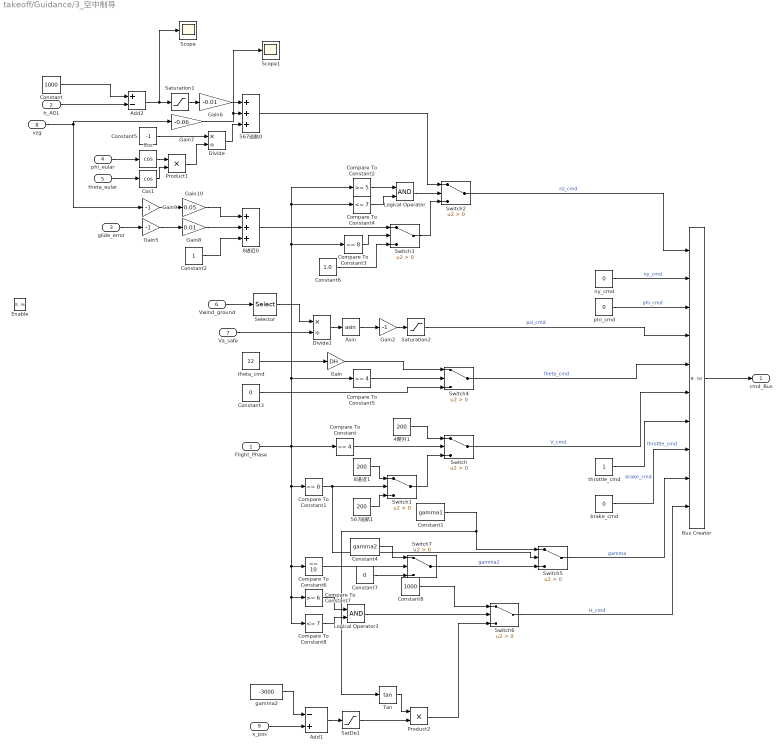
== system takeoff/Guidance/3_空中制导 ==
  Flight_Phase : Inport
  h_AGL : Inport  Port=2
  glide_error : Inport  Port=3
  phi_eular : Inport  Port=4
  theta_eular : Inport  Port=5
  Vwind_ground : Inport  Port=6
  Va_safe : Inport  Port=7
  vzg : Inport  Port=8
  x_pos : Inport  Port=9
  Enable : EnablePort
  4爬升1 : Constant  Value=200
  567巡航0 : Sum  Inputs=+++
  567巡航1 : Constant  Value=200
  8进近0 : Sum  Inputs=+++
  8进近1 : Constant  Value=200
  Add1 : Sum  Inputs=-+
  Add2 : Sum  Inputs=+-
  Asin : Trigonometry  Operator=asin
  Bus Creator : BusCreator  Inputs=10
  Compare To Constant : simulink/Logic and Bit Operations/Compare To Constant  relop===  const=4  OutDataTypeStr=boolean
  Compare To Constant1 : simulink/Logic and Bit Operations/Compare To Constant  relop===  const=8  OutDataTypeStr=boolean
  Compare To Constant2 : simulink/Logic and Bit Operations/Compare To Constant  relop=>=  const=5  OutDataTypeStr=boolean
  Compare To Constant3 : simulink/Logic and Bit Operations/Compare To Constant  relop===  const=8  OutDataTypeStr=boolean
  Compare To Constant4 : simulink/Logic and Bit Operations/Compare To Constant  relop=<=  const=7  OutDataTypeStr=boolean
  Compare To Constant5 : simulink/Logic and Bit Operations/Compare To Constant  relop===  const=4  OutDataTypeStr=boolean
  Compare To Constant6 : simulink/Logic and Bit Operations/Compare To Constant  relop===  const=10  OutDataTypeStr=boolean
  Compare To Constant7 : simulink/Logic and Bit Operations/Compare To Constant  relop=>=  const=6  OutDataTypeStr=boolean
  Compare To Constant8 : simulink/Logic and Bit Operations/Compare To Constant  relop=<=  const=7  OutDataTypeStr=boolean
  Constant : Constant  Value=1000
  Constant1 : Constant  Value=gamma1
  Constant2 : Constant
  Constant3 : Constant  Value=0
  Constant4 : Constant  Value=gamma2
  Constant5 : Constant  Value=-1
  Constant6 : Constant  Value=1.0
  Constant7 : Constant  Value=0
  Constant8 : Constant  Value=1000
  Cos : Trigonometry  Operator=cos
  Cos1 : Trigonometry  Operator=cos
  Divide : Product  Inputs=*/
  Divide1 : Product  Inputs=*/
  Gain : Gain  Gain=DH
  Gain10 : Gain  Gain=0.05
  Gain2 : Gain  Gain=-1
  Gain5 : Gain  Gain=-1
  Gain6 : Gain  Gain=-0.01
  Gain7 : Gain  Gain=-0.06
  Gain8 : Gain  Gain=0.01
  Gain9 : Gain  Gain=-1
  Logical Operator : Logic  AllPortsSameDT=off  OutDataTypeStr=boolean
  Logical Operator3 : Logic  AllPortsSameDT=off  OutDataTypeStr=boolean
  Product1 : Product
  Product2 : Product
  SatDe1 : Saturate  UpperLimit=8000  LowerLimit=-8000
  Saturation1 : Saturate  UpperLimit=100  LowerLimit=-100
  Saturation2 : Saturate  UpperLimit=10*DH  LowerLimit=-10*DH
  Scope : Scope
      settings: ActiveDisplayYMinimum=-643.50538  ActiveDisplayYMaximum=1162.25948  DataLoggingVariableName=ScopeData2
  Scope1 : Scope
      settings: ActiveDisplayYMinimum=-1.38659  ActiveDisplayYMaximum=2.42946  DataLoggingVariableName=ScopeData3
  Selector : Selector  InputPortWidth=3  IndexOptions=Index vector (dialog)  Indices=2  OutputSizes=1
  Switch{,1..7} (8 alike) : Switch  Criteria=u2 > Threshold  SaturateOnIntegerOverflow=off  InputSameDT=off
  Tan : Trigonometry  Operator=tan
  brake_cmd : Constant  Value=0
  gamma2 : Constant  Value=-3000
  ny_cmd : Constant  Value=0
  phi_cmd : Constant  Value=0
  theta_cmd : Constant  Value=12
  throttle_cmd : Constant
  cmd_Bus : Outport
  wires:
  brake_cmd/1 -> Bus Creator/8  "brake_cmd"
  Saturation2/1 -> Bus Creator/4  "psi_cmd"
  Switch/1 -> Bus Creator/6  "V_cmd"
  Bus Creator/1 -> cmd_Bus/1
  Compare To Constant/1 -> Switch/2
  4爬升1/1 -> Switch/1
  Switch1/1 -> Switch/3
  Compare To Constant1/1 -> Switch1/2, Switch5/2
  8进近1/1 -> Switch1/1
  567巡航1/1 -> Switch1/3
  vzg/1 -> Gain7/1, Gain9/1
  Gain6/1 -> 567巡航0/1
  Gain7/1 -> Scope1/1, 567巡航0/2
  h_AGL/1 -> Add2/2
  Constant/1 -> Add2/1
  glide_error/1 -> Gain5/1
  Gain5/1 -> Gain8/1
  Gain8/1 -> 8进近0/2
  Gain9/1 -> Gain10/1
  Gain10/1 -> 8进近0/1
  Constant2/1 -> 8进近0/3
  Compare To Constant3/1 -> Switch3/2
  Flight_Phase/1 -> Compare To Constant2/1, Compare To Constant4/1, Compare To Constant3/1, Compare To Constant5/1, Compare To Constant8/1, Compare To Constant7/1, Compare To Constant6/1, Compare To Constant1/1, Compare To Constant/1
  throttle_cmd/1 -> Bus Creator/7  "throttle_cmd"
  Compare To Constant2/1 -> Logical Operator/1
  Compare To Constant4/1 -> Logical Operator/2
  Logical Operator/1 -> Switch2/2
  567巡航0/1 -> Switch2/1
  Switch3/1 -> Switch2/3
  Constant6/1 -> Switch3/3
  8进近0/1 -> Switch3/1
  Switch2/1 -> Bus Creator/1  "nz_cmd"
  Compare To Constant5/1 -> Switch4/2
  Switch4/1 -> Bus Creator/5  "theta_cmd"
  Constant3/1 -> Switch4/3
  theta_cmd/1 -> Gain/1
  phi_eular/1 -> Cos/1
  Cos/1 -> Product1/1
  Divide/1 -> 567巡航0/3
  Constant5/1 -> Divide/1
  Product1/1 -> Divide/2
  Cos1/1 -> Product1/2
  Asin/1 -> Gain2/1
  Gain2/1 -> Saturation2/1
  Divide1/1 -> Asin/1
  Selector/1 -> Divide1/1
  Va_safe/1 -> Divide1/2
  ny_cmd/1 -> Bus Creator/2  "ny_cmd"
  phi_cmd/1 -> Bus Creator/3  "phi_cmd"
  Gain/1 -> Switch4/1
  theta_eular/1 -> Cos1/1
  Vwind_ground/1 -> Selector/1
  Saturation1/1 -> Gain6/1
  Add2/1 -> Scope/1, Saturation1/1
  Switch5/1 -> Bus Creator/9  "gamma"
  Switch6/1 -> Bus Creator/10  "H_cmd"
  Compare To Constant6/1 -> Switch7/2
  Constant4/1 -> Switch7/1
  Constant7/1 -> Switch7/3
  Compare To Constant7/1 -> Logical Operator3/1
  Compare To Constant8/1 -> Logical Operator3/2
  Logical Operator3/1 -> Switch6/2
  Constant8/1 -> Switch6/1
  Constant1/1 -> Tan/1, Switch5/1
  Tan/1 -> Product2/1
  SatDe1/1 -> Product2/2
  Add1/1 -> SatDe1/1
  x_pos/1 -> Add1/2
  gamma2/1 -> Add1/1
  Product2/1 -> Switch6/3
  Switch7/1 -> Switch5/3  "gamma2"
